simulink model "Equilibrium_point"  (R2023b)
settings: Solver=VariableStepAuto  StartTime=0.0  StopTime=100  RelTol=1e-3
settings Model: Creator=nasir  LastModifiedBy=nasir

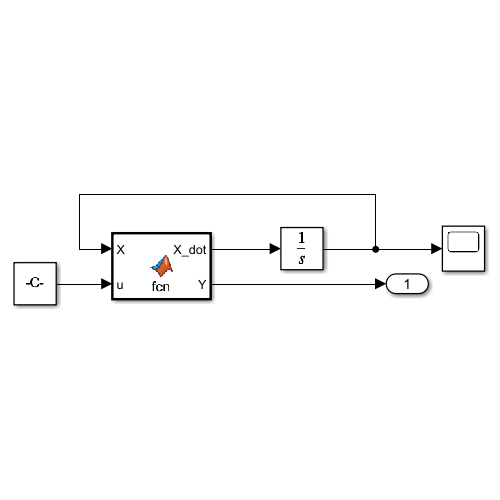
[thumbnail: Simulink's stored preview of the top-level diagram]
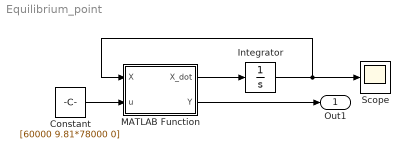
== system Equilibrium_point ==
  Constant : Constant  Value=[60000 9.81*78000 0]
  Integrator : Integrator  InitialCondition=[800/3.6 0 60000/(9.81*78000) 0]
  MATLAB Function : MATLAB Function  TreatAsAtomicUnit=on
  Scope : Scope
  Out1 : Outport
  wires:
  Constant/1 -> MATLAB Function/2(u)
  MATLAB Function/1(X_dot) -> Integrator/1
  Integrator/1 -> MATLAB Function/1(X), Scope/1
  MATLAB Function/2(Y) -> Out1/1

== matlab function Equilibrium_point/MATLAB Function ==
  data: X input; u input; X_dot output; Y output
function [X_dot, Y]= fcn(X, u)
%#codegen
m = 78000;
Iy = 9*10e6;
g = 9.81;


X_dot = [u(1)/m - g*sin(X(3))-X(4)*X(2);
    u(2)/m - g*cos(X(3))+X(4)*X(1);
    X(4);
    u(3)/Iy];

Y = [X(3);
    X(4)];
